simulink library "inp"  (R2021b)
settings: Solver=VariableStepAuto  StartTime=0.0  StopTime=10.0  RelTol=1e-3
undefined symbols (not defined in the file): C_TASK_5MS_S, FALSE, KINP_AcoreReadyToSlp_flg_ovrdflg, KINP_AcoreReadyToSlp_flg_ovrdval, KINP_AllowMovThd_OTA_enum_ovrdflg, KINP_AllowMovThd_OTA_enum_ovrdval, KINP_APSAngleTarget_Deg_ovrdflg, KINP_APSAngleTarget_Deg_ovrdval, KINP_APSDecReq_mps2_ovrdflg, KINP_APSDecReq_mps2_ovrdval, KINP_APSDecReqA_flg_ovrdflg, KINP_APSDecReqA_flg_ovrdval, KINP_APSDFLL_cm_ovrdflg, KINP_APSDFLL_cm_ovrdval, KINP_APSDFLR_cm_ovrdflg, KINP_APSDFLR_cm_ovrdval, KINP_APSDRLL_cm_ovrdflg, KINP_APSDRLL_cm_ovrdval, KINP_APSDRLR_cm_ovrdflg, KINP_APSDRLR_cm_ovrdval, KINP_APSExitCondition_enum_ovrdflg, KINP_APSExitCondition_enum_ovrdval, KINP_APSHWVer_enum_ovrdflg, KINP_APSHWVer_enum_ovrdval, KINP_APSProgressPCT_pct_ovrdflg, KINP_APSProgressPCT_pct_ovrdval, KINP_APSReq_enum_ovrdflg, KINP_APSReq_enum_ovrdval, KINP_APSRQDisplay_enum_ovrdflg, KINP_APSRQDisplay_enum_ovrdval, KINP_APSRqEPASCtrl_flg_ovrdflg, KINP_APSRqEPASCtrl_flg_ovrdval, KINP_APSShiftPosnReq_enum_ovrdval, KINP_APSShiftPosnReq_enum_ovrflg, KINP_APSSpeedCMD_kph_ovrdval, KINP_APSSpeedCMD_kph_ovrflg, KINP_APSStaSystem_enum_ovrdflg, KINP_APSStaSystem_enum_ovrdval, KINP_APSSWVer_enum_ovrdflg, KINP_APSSWVer_enum_ovrdval, KINP_APSVMCReqA_flg_ovrdval, KINP_APSVMCReqA_flg_ovrflg, KINP_APSVRqEPASCtrl_flg_ovrdflg, KINP_APSVRqEPASCtrl_flg_ovrdval, KINP_AuxBattVolmV_mV_ovrdflg, KINP_AuxBattVolmV_mV_ovrdval, KINP_CAASSta_enum_ovrdflg, KINP_CAASSta_enum_ovrdval, KINP_CAASVMCReqA_flg_ovrdval, KINP_CAASVMCReqA_flg_ovrflg, KINP_Chime_enum_ovrdflg, KINP_Chime_enum_ovrdval, KINP_ClearDTCcmd_flg_ovrdflg, KINP_ClearDTCcmd_flg_ovrdval, KINP_EvccAplusPwrUpReq_flg_ovrdflg, KINP_EvccAplusPwrUpReq_flg_ovrdval, KINP_LFID_raw_ovrdval, KINP_LFID_raw_ovrflg, KINP_LRID_raw_ovrdval, KINP_MemOffsetAccX_raw16_ovrdflg ... (+118)
libraries: FVT_lib x503, hcu_lib x1
(part 8 of 16)

== system inp/INP/CAN1/SignalCheck/EMC1_EM1 ==
  BHAL_outputs : Inport
  inp_CanValid_bus : Inport  Port=2
  EM1CS : FVT_lib/inp/can_signal_template  SystemSampleTime=-1  VariantActivationTime=update diagram  Latency=0  AutoFrameSizeCalculation=off
      link override defval: Value=KINP_EM1CS_enum_defval
      link override ovrdflg: Value=KINP_EM1CS_enum_ovrdflg
      link override ovrdval: Value=KINP_EM1CS_enum_ovrdval
  EM1Cnt : FVT_lib/inp/can_signal_template  SystemSampleTime=-1  VariantActivationTime=update diagram  Latency=0  AutoFrameSizeCalculation=off
      link override defval: Value=KINP_EM1Cnt_enum_defval
      link override ovrdflg: Value=KINP_EM1Cnt_enum_ovrdflg
      link override ovrdval: Value=KINP_EM1Cnt_enum_ovrdval
  EM1OvrCtrlMBrk : FVT_lib/inp/can_signal_template  SystemSampleTime=-1  VariantActivationTime=update diagram  Latency=0  AutoFrameSizeCalculation=off
      link override defval: Value=KINP_EM1OvrCtrlMBrk_enum_defval
      link override ovrdflg: Value=KINP_EM1OvrCtrlMBrk_enum_ovrdflg
      link override ovrdval: Value=KINP_EM1OvrCtrlMBrk_enum_ovrdval
  EM1OvrCtrlMDriv : FVT_lib/inp/can_signal_template  SystemSampleTime=-1  VariantActivationTime=update diagram  Latency=0  AutoFrameSizeCalculation=off
      link override defval: Value=KINP_EM1OvrCtrlMDriv_enum_defval
      link override ovrdflg: Value=KINP_EM1OvrCtrlMDriv_enum_ovrdflg
      link override ovrdval: Value=KINP_EM1OvrCtrlMDriv_enum_ovrdval
  EM1OvrCtrlMPriBrk : FVT_lib/inp/can_signal_template  SystemSampleTime=-1  VariantActivationTime=update diagram  Latency=0  AutoFrameSizeCalculation=off
      link override defval: Value=KINP_EM1OvrCtrlMPriBrk_enum_defval
      link override ovrdflg: Value=KINP_EM1OvrCtrlMPriBrk_enum_ovrdflg
      link override ovrdval: Value=KINP_EM1OvrCtrlMPriBrk_enum_ovrdval
  EM1OvrCtrlMPriDriv : FVT_lib/inp/can_signal_template  SystemSampleTime=-1  VariantActivationTime=update diagram  Latency=0  AutoFrameSizeCalculation=off
      link override defval: Value=KINP_EM1OvrCtrlMPriDriv_enum_defval
      link override ovrdflg: Value=KINP_EM1OvrCtrlMPriDriv_enum_ovrdflg
      link override ovrdval: Value=KINP_EM1OvrCtrlMPriDriv_enum_ovrdval
  EM1ReqTorqHRlsBrk : FVT_lib/inp/can_signal_template  SystemSampleTime=-1  VariantActivationTime=update diagram  Latency=0  AutoFrameSizeCalculation=off
      link override defval: Value=KINP_EM1ReqTorqHRlsBrk_pct_defval
      link override ovrdflg: Value=KINP_EM1ReqTorqHRlsBrk_pct_ovrdflg
      link override ovrdval: Value=KINP_EM1ReqTorqHRlsBrk_pct_ovrdval
  EM1ReqTorqHRlsDri : FVT_lib/inp/can_signal_template  SystemSampleTime=-1  VariantActivationTime=update diagram  Latency=0  AutoFrameSizeCalculation=off
      link override defval: Value=KINP_EM1ReqTorqHRlsDri_pct_defval
      link override ovrdflg: Value=KINP_EM1ReqTorqHRlsDri_pct_ovrdflg
      link override ovrdval: Value=KINP_EM1ReqTorqHRlsDri_pct_ovrdval
  EM1ReqTorqLimBrk : FVT_lib/inp/can_signal_template  SystemSampleTime=-1  VariantActivationTime=update diagram  Latency=0  AutoFrameSizeCalculation=off
      link override defval: Value=KINP_EM1ReqTorqLimBrk_pct_defval
      link override ovrdflg: Value=KINP_EM1ReqTorqLimBrk_pct_ovrdflg
      link override ovrdval: Value=KINP_EM1ReqTorqLimBrk_pct_ovrdval
  EM1ReqTorqLimDriv : FVT_lib/inp/can_signal_template  SystemSampleTime=-1  VariantActivationTime=update diagram  Latency=0  AutoFrameSizeCalculation=off
      link override defval: Value=KINP_EM1ReqTorqLimDriv_pct_defval
      link override ovrdflg: Value=KINP_EM1ReqTorqLimDriv_pct_ovrdflg
      link override ovrdval: Value=KINP_EM1ReqTorqLimDriv_pct_ovrdval
  Terminator_{1..10} (10 alike) : Terminator
  True_VHAL_EM1CS_enum : Constant  Value=TRUE  OutDataTypeStr=boolean
  True_VHAL_EM1Cnt_enum : Constant  Value=TRUE  OutDataTypeStr=boolean
  True_VHAL_EM1OvrCtrlMBrk_enum : Constant  Value=TRUE  OutDataTypeStr=boolean
  True_VHAL_EM1OvrCtrlMDriv_enum : Constant  Value=TRUE  OutDataTypeStr=boolean
  True_VHAL_EM1OvrCtrlMPriBrk_enum : Constant  Value=TRUE  OutDataTypeStr=boolean
  True_VHAL_EM1OvrCtrlMPriDriv_enum : Constant  Value=TRUE  OutDataTypeStr=boolean
  True_VHAL_EM1ReqTorqHRlsBrk_pct : Constant  Value=TRUE  OutDataTypeStr=boolean
  True_VHAL_EM1ReqTorqHRlsDri_pct : Constant  Value=TRUE  OutDataTypeStr=boolean
  True_VHAL_EM1ReqTorqLimBrk_pct : Constant  Value=TRUE  OutDataTypeStr=boolean
  True_VHAL_EM1ReqTorqLimDriv_pct : Constant  Value=TRUE  OutDataTypeStr=boolean
  slr1_{1..10} (10 alike) : BusSelector  OutputSignals=VINP_CANMsgValidEMC1EM1_flg
  slr_VHAL_EM1CS_enum : BusSelector  OutputSignals=VHAL_EM1CS_enum
  slr_VHAL_EM1Cnt_enum : BusSelector  OutputSignals=VHAL_EM1Cnt_enum
  slr_VHAL_EM1OvrCtrlMBrk_enum : BusSelector  OutputSignals=VHAL_EM1OvrCtrlMBrk_enum
  slr_VHAL_EM1OvrCtrlMDriv_enum : BusSelector  OutputSignals=VHAL_EM1OvrCtrlMDriv_enum
  slr_VHAL_EM1OvrCtrlMPriBrk_enum : BusSelector  OutputSignals=VHAL_EM1OvrCtrlMPriBrk_enum
  slr_VHAL_EM1OvrCtrlMPriDriv_enum : BusSelector  OutputSignals=VHAL_EM1OvrCtrlMPriDriv_enum
  slr_VHAL_EM1ReqTorqHRlsBrk_pct : BusSelector  OutputSignals=VHAL_EM1ReqTorqHRlsBrk_pct
  slr_VHAL_EM1ReqTorqHRlsDri_pct : BusSelector  OutputSignals=VHAL_EM1ReqTorqHRlsDri_pct
  slr_VHAL_EM1ReqTorqLimBrk_pct : BusSelector  OutputSignals=VHAL_EM1ReqTorqLimBrk_pct
  slr_VHAL_EM1ReqTorqLimDriv_pct : BusSelector  OutputSignals=VHAL_EM1ReqTorqLimDriv_pct
  VINP_EM1CS_enum : Outport
  VINP_EM1Cnt_enum : Outport  Port=2
  VINP_EM1OvrCtrlMBrk_enum : Outport  Port=3
  VINP_EM1OvrCtrlMDriv_enum : Outport  Port=4
  VINP_EM1OvrCtrlMPriBrk_enum : Outport  Port=5
  VINP_EM1OvrCtrlMPriDriv_enum : Outport  Port=6
  VINP_EM1ReqTorqHRlsBrk_pct : Outport  Port=7
  VINP_EM1ReqTorqHRlsDri_pct : Outport  Port=8
  VINP_EM1ReqTorqLimBrk_pct : Outport  Port=9
  VINP_EM1ReqTorqLimDriv_pct : Outport  Port=10
  wires:
  BHAL_outputs/1 -> [BHAL_outputs]
  inp_CanValid_bus/1 -> [inp_CanValid_bus]
  [BHAL_outputs] -> slr_VHAL_EM1CS_enum/1
  slr_VHAL_EM1CS_enum/1 -> EM1CS/1  "<VHAL_EM1CS_enum>"
  True_VHAL_EM1CS_enum/1 -> EM1CS/2
  [inp_CanValid_bus] -> slr1_1/1
  slr1_1/1 -> EM1CS/3  "<VINP_CANMsgValidEMC1EM1_flg>"
  EM1CS/1 -> VINP_EM1CS_enum/1  "VINP_EM1CS_enum"
  EM1CS/2 -> Terminator_1/1
  [BHAL_outputs] -> slr_VHAL_EM1Cnt_enum/1
  slr_VHAL_EM1Cnt_enum/1 -> EM1Cnt/1  "<VHAL_EM1Cnt_enum>"
  True_VHAL_EM1Cnt_enum/1 -> EM1Cnt/2
  [inp_CanValid_bus] -> slr1_2/1
  slr1_2/1 -> EM1Cnt/3  "<VINP_CANMsgValidEMC1EM1_flg>"
  EM1Cnt/1 -> VINP_EM1Cnt_enum/1  "VINP_EM1Cnt_enum"
  EM1Cnt/2 -> Terminator_2/1
  [BHAL_outputs] -> slr_VHAL_EM1OvrCtrlMBrk_enum/1
  slr_VHAL_EM1OvrCtrlMBrk_enum/1 -> EM1OvrCtrlMBrk/1  "<VHAL_EM1OvrCtrlMBrk_enum>"
  True_VHAL_EM1OvrCtrlMBrk_enum/1 -> EM1OvrCtrlMBrk/2
  [inp_CanValid_bus] -> slr1_3/1
  slr1_3/1 -> EM1OvrCtrlMBrk/3  "<VINP_CANMsgValidEMC1EM1_flg>"
  EM1OvrCtrlMBrk/1 -> VINP_EM1OvrCtrlMBrk_enum/1  "VINP_EM1OvrCtrlMBrk_enum"
  EM1OvrCtrlMBrk/2 -> Terminator_3/1
  [BHAL_outputs] -> slr_VHAL_EM1OvrCtrlMDriv_enum/1
  slr_VHAL_EM1OvrCtrlMDriv_enum/1 -> EM1OvrCtrlMDriv/1  "<VHAL_EM1OvrCtrlMDriv_enum>"
  True_VHAL_EM1OvrCtrlMDriv_enum/1 -> EM1OvrCtrlMDriv/2
  [inp_CanValid_bus] -> slr1_4/1
  slr1_4/1 -> EM1OvrCtrlMDriv/3  "<VINP_CANMsgValidEMC1EM1_flg>"
  EM1OvrCtrlMDriv/1 -> VINP_EM1OvrCtrlMDriv_enum/1  "VINP_EM1OvrCtrlMDriv_enum"
  EM1OvrCtrlMDriv/2 -> Terminator_4/1
  [BHAL_outputs] -> slr_VHAL_EM1OvrCtrlMPriBrk_enum/1
  slr_VHAL_EM1OvrCtrlMPriBrk_enum/1 -> EM1OvrCtrlMPriBrk/1  "<VHAL_EM1OvrCtrlMPriBrk_enum>"
  True_VHAL_EM1OvrCtrlMPriBrk_enum/1 -> EM1OvrCtrlMPriBrk/2
  [inp_CanValid_bus] -> slr1_5/1
  slr1_5/1 -> EM1OvrCtrlMPriBrk/3  "<VINP_CANMsgValidEMC1EM1_flg>"
  EM1OvrCtrlMPriBrk/1 -> VINP_EM1OvrCtrlMPriBrk_enum/1  "VINP_EM1OvrCtrlMPriBrk_enum"
  EM1OvrCtrlMPriBrk/2 -> Terminator_5/1
  [BHAL_outputs] -> slr_VHAL_EM1OvrCtrlMPriDriv_enum/1
  slr_VHAL_EM1OvrCtrlMPriDriv_enum/1 -> EM1OvrCtrlMPriDriv/1  "<VHAL_EM1OvrCtrlMPriDriv_enum>"
  True_VHAL_EM1OvrCtrlMPriDriv_enum/1 -> EM1OvrCtrlMPriDriv/2
  [inp_CanValid_bus] -> slr1_6/1
  slr1_6/1 -> EM1OvrCtrlMPriDriv/3  "<VINP_CANMsgValidEMC1EM1_flg>"
  EM1OvrCtrlMPriDriv/1 -> VINP_EM1OvrCtrlMPriDriv_enum/1  "VINP_EM1OvrCtrlMPriDriv_enum"
  EM1OvrCtrlMPriDriv/2 -> Terminator_6/1
  [BHAL_outputs] -> slr_VHAL_EM1ReqTorqHRlsBrk_pct/1
  slr_VHAL_EM1ReqTorqHRlsBrk_pct/1 -> EM1ReqTorqHRlsBrk/1  "<VHAL_EM1ReqTorqHRlsBrk_pct>"
  True_VHAL_EM1ReqTorqHRlsBrk_pct/1 -> EM1ReqTorqHRlsBrk/2
  [inp_CanValid_bus] -> slr1_7/1
  slr1_7/1 -> EM1ReqTorqHRlsBrk/3  "<VINP_CANMsgValidEMC1EM1_flg>"
  EM1ReqTorqHRlsBrk/1 -> VINP_EM1ReqTorqHRlsBrk_pct/1  "VINP_EM1ReqTorqHRlsBrk_pct"
  EM1ReqTorqHRlsBrk/2 -> Terminator_7/1
  [BHAL_outputs] -> slr_VHAL_EM1ReqTorqHRlsDri_pct/1
  slr_VHAL_EM1ReqTorqHRlsDri_pct/1 -> EM1ReqTorqHRlsDri/1  "<VHAL_EM1ReqTorqHRlsDri_pct>"
  True_VHAL_EM1ReqTorqHRlsDri_pct/1 -> EM1ReqTorqHRlsDri/2
  [inp_CanValid_bus] -> slr1_8/1
  slr1_8/1 -> EM1ReqTorqHRlsDri/3  "<VINP_CANMsgValidEMC1EM1_flg>"
  EM1ReqTorqHRlsDri/1 -> VINP_EM1ReqTorqHRlsDri_pct/1  "VINP_EM1ReqTorqHRlsDri_pct"
  EM1ReqTorqHRlsDri/2 -> Terminator_8/1
  [BHAL_outputs] -> slr_VHAL_EM1ReqTorqLimBrk_pct/1
  slr_VHAL_EM1ReqTorqLimBrk_pct/1 -> EM1ReqTorqLimBrk/1  "<VHAL_EM1ReqTorqLimBrk_pct>"
  True_VHAL_EM1ReqTorqLimBrk_pct/1 -> EM1ReqTorqLimBrk/2
  [inp_CanValid_bus] -> slr1_9/1
  slr1_9/1 -> EM1ReqTorqLimBrk/3  "<VINP_CANMsgValidEMC1EM1_flg>"
  EM1ReqTorqLimBrk/1 -> VINP_EM1ReqTorqLimBrk_pct/1  "VINP_EM1ReqTorqLimBrk_pct"
  EM1ReqTorqLimBrk/2 -> Terminator_9/1
  [BHAL_outputs] -> slr_VHAL_EM1ReqTorqLimDriv_pct/1
  slr_VHAL_EM1ReqTorqLimDriv_pct/1 -> EM1ReqTorqLimDriv/1  "<VHAL_EM1ReqTorqLimDriv_pct>"
  True_VHAL_EM1ReqTorqLimDriv_pct/1 -> EM1ReqTorqLimDriv/2
  [inp_CanValid_bus] -> slr1_10/1
  slr1_10/1 -> EM1ReqTorqLimDriv/3  "<VINP_CANMsgValidEMC1EM1_flg>"
  EM1ReqTorqLimDriv/1 -> VINP_EM1ReqTorqLimDriv_pct/1  "VINP_EM1ReqTorqLimDriv_pct"
  EM1ReqTorqLimDriv/2 -> Terminator_10/1

== system inp/INP/CAN1/SignalCheck/EPB1 ==
  BHAL_outputs : Inport
  inp_CanValid_bus : Inport  Port=2
  EPBParkingBrakeSta : FVT_lib/inp/can_signal_template  SystemSampleTime=-1  VariantActivationTime=update diagram  Latency=0  AutoFrameSizeCalculation=off
      link override defval: Value=KINP_EPBParkingBrakeSta_enum_defval
      link override ovrdflg: Value=KINP_EPBParkingBrakeSta_enum_ovrdflg
      link override ovrdval: Value=KINP_EPBParkingBrakeSta_enum_ovrdval
  Terminator_1 : Terminator
  True_VHAL_EPBParkingBrakeSta_enum : Constant  Value=TRUE  OutDataTypeStr=boolean
  slr1_1 : BusSelector  OutputSignals=VINP_CANMsgValidEPB1_flg
  slr_VHAL_EPBParkingBrakeSta_enum : BusSelector  OutputSignals=VHAL_EPBParkingBrakeSta_enum
  VINP_EPBParkingBrakeSta_enum : Outport
  wires:
  BHAL_outputs/1 -> [BHAL_outputs]
  inp_CanValid_bus/1 -> [inp_CanValid_bus]
  [BHAL_outputs] -> slr_VHAL_EPBParkingBrakeSta_enum/1
  slr_VHAL_EPBParkingBrakeSta_enum/1 -> EPBParkingBrakeSta/1  "<VHAL_EPBParkingBrakeSta_enum>"
  True_VHAL_EPBParkingBrakeSta_enum/1 -> EPBParkingBrakeSta/2
  [inp_CanValid_bus] -> slr1_1/1
  slr1_1/1 -> EPBParkingBrakeSta/3  "<VINP_CANMsgValidEPB1_flg>"
  EPBParkingBrakeSta/1 -> VINP_EPBParkingBrakeSta_enum/1  "VINP_EPBParkingBrakeSta_enum"
  EPBParkingBrakeSta/2 -> Terminator_1/1

== system inp/INP/CAN1/SignalCheck/PDU_Status_1 ==
  BHAL_outputs : Inport
  inp_CanValid_bus : Inport  Port=2
  PDUDCDCRlySta : FVT_lib/inp/can_signal_template  SystemSampleTime=-1  VariantActivationTime=update diagram  Latency=0  AutoFrameSizeCalculation=off
      link override defval: Value=KINP_PDUDCDCRlySta_enum_defval
      link override ovrdflg: Value=KINP_PDUDCDCRlySta_enum_ovrdflg
      link override ovrdval: Value=KINP_PDUDCDCRlySta_enum_ovrdval
  PDUEACRlySta : FVT_lib/inp/can_signal_template  SystemSampleTime=-1  VariantActivationTime=update diagram  Latency=0  AutoFrameSizeCalculation=off
      link override defval: Value=KINP_PDUEACRlySta_enum_defval
      link override ovrdflg: Value=KINP_PDUEACRlySta_enum_ovrdflg
      link override ovrdval: Value=KINP_PDUEACRlySta_enum_ovrdval
  PDUEHPSRlySta : FVT_lib/inp/can_signal_template  SystemSampleTime=-1  VariantActivationTime=update diagram  Latency=0  AutoFrameSizeCalculation=off
      link override defval: Value=KINP_PDUEHPSRlySta_enum_defval
      link override ovrdflg: Value=KINP_PDUEHPSRlySta_enum_ovrdflg
      link override ovrdval: Value=KINP_PDUEHPSRlySta_enum_ovrdval
  PDUSelfChkSta : FVT_lib/inp/can_signal_template  SystemSampleTime=-1  VariantActivationTime=update diagram  Latency=0  AutoFrameSizeCalculation=off
      link override defval: Value=KINP_PDUSelfChkSta_enum_defval
      link override ovrdflg: Value=KINP_PDUSelfChkSta_enum_ovrdflg
      link override ovrdval: Value=KINP_PDUSelfChkSta_enum_ovrdval
  Terminator_{1..4} (4 alike) : Terminator
  True_VHAL_PDUDCDCRlySta_enum : Constant  Value=TRUE  OutDataTypeStr=boolean
  True_VHAL_PDUEACRlySta_enum : Constant  Value=TRUE  OutDataTypeStr=boolean
  True_VHAL_PDUEHPSRlySta_enum : Constant  Value=TRUE  OutDataTypeStr=boolean
  True_VHAL_PDUSelfChkSta_enum : Constant  Value=TRUE  OutDataTypeStr=boolean
  slr1_{1..4} (4 alike) : BusSelector  OutputSignals=VINP_CANMsgValidPDUStatus1_flg
  slr_VHAL_PDUDCDCRlySta_enum : BusSelector  OutputSignals=VHAL_PDUDCDCRlySta_enum
  slr_VHAL_PDUEACRlySta_enum : BusSelector  OutputSignals=VHAL_PDUEACRlySta_enum
  slr_VHAL_PDUEHPSRlySta_enum : BusSelector  OutputSignals=VHAL_PDUEHPSRlySta_enum
  slr_VHAL_PDUSelfChkSta_enum : BusSelector  OutputSignals=VHAL_PDUSelfChkSta_enum
  VINP_PDUDCDCRlySta_enum : Outport
  VINP_PDUEACRlySta_enum : Outport  Port=2
  VINP_PDUEHPSRlySta_enum : Outport  Port=3
  VINP_PDUSelfChkSta_enum : Outport  Port=4
  wires:
  BHAL_outputs/1 -> [BHAL_outputs]
  inp_CanValid_bus/1 -> [inp_CanValid_bus]
  [BHAL_outputs] -> slr_VHAL_PDUDCDCRlySta_enum/1
  slr_VHAL_PDUDCDCRlySta_enum/1 -> PDUDCDCRlySta/1  "<VHAL_PDUDCDCRlySta_enum>"
  True_VHAL_PDUDCDCRlySta_enum/1 -> PDUDCDCRlySta/2
  [inp_CanValid_bus] -> slr1_1/1
  slr1_1/1 -> PDUDCDCRlySta/3  "<VINP_CANMsgValidPDUStatus1_flg>"
  PDUDCDCRlySta/1 -> VINP_PDUDCDCRlySta_enum/1  "VINP_PDUDCDCRlySta_enum"
  PDUDCDCRlySta/2 -> Terminator_1/1
  [BHAL_outputs] -> slr_VHAL_PDUEACRlySta_enum/1
  slr_VHAL_PDUEACRlySta_enum/1 -> PDUEACRlySta/1  "<VHAL_PDUEACRlySta_enum>"
  True_VHAL_PDUEACRlySta_enum/1 -> PDUEACRlySta/2
  [inp_CanValid_bus] -> slr1_2/1
  slr1_2/1 -> PDUEACRlySta/3  "<VINP_CANMsgValidPDUStatus1_flg>"
  PDUEACRlySta/1 -> VINP_PDUEACRlySta_enum/1  "VINP_PDUEACRlySta_enum"
  PDUEACRlySta/2 -> Terminator_2/1
  [BHAL_outputs] -> slr_VHAL_PDUEHPSRlySta_enum/1
  slr_VHAL_PDUEHPSRlySta_enum/1 -> PDUEHPSRlySta/1  "<VHAL_PDUEHPSRlySta_enum>"
  True_VHAL_PDUEHPSRlySta_enum/1 -> PDUEHPSRlySta/2
  [inp_CanValid_bus] -> slr1_3/1
  slr1_3/1 -> PDUEHPSRlySta/3  "<VINP_CANMsgValidPDUStatus1_flg>"
  PDUEHPSRlySta/1 -> VINP_PDUEHPSRlySta_enum/1  "VINP_PDUEHPSRlySta_enum"
  PDUEHPSRlySta/2 -> Terminator_3/1
  [BHAL_outputs] -> slr_VHAL_PDUSelfChkSta_enum/1
  slr_VHAL_PDUSelfChkSta_enum/1 -> PDUSelfChkSta/1  "<VHAL_PDUSelfChkSta_enum>"
  True_VHAL_PDUSelfChkSta_enum/1 -> PDUSelfChkSta/2
  [inp_CanValid_bus] -> slr1_4/1
  slr1_4/1 -> PDUSelfChkSta/3  "<VINP_CANMsgValidPDUStatus1_flg>"
  PDUSelfChkSta/1 -> VINP_PDUSelfChkSta_enum/1  "VINP_PDUSelfChkSta_enum"
  PDUSelfChkSta/2 -> Terminator_4/1

== system inp/INP/CAN2/SignalCheck/IVI1 ==
  BHAL_outputs : Inport
  inp_CanValid_bus : Inport  Port=2
  AmbLighLowBatAlertSW : FVT_lib/inp/can_signal_template  SystemSampleTime=-1  VariantActivationTime=update diagram  Latency=0  AutoFrameSizeCalculation=off
      link override defval: Value=KINP_AmbLighLowBatAlertSW_flg_defval
      link override ovrdflg: Value=KINP_AmbLighLowBatAlertSW_flg_ovrdflg
      link override ovrdval: Value=KINP_AmbLighLowBatAlertSW_flg_ovrdval
  AmbLighSafetyAlertSW : FVT_lib/inp/can_signal_template  SystemSampleTime=-1  VariantActivationTime=update diagram  Latency=0  AutoFrameSizeCalculation=off
      link override defval: Value=KINP_AmbLighSafetyAlertSW_flg_defval
      link override ovrdflg: Value=KINP_AmbLighSafetyAlertSW_flg_ovrdflg
      link override ovrdval: Value=KINP_AmbLighSafetyAlertSW_flg_ovrdval
  AmbLightColorSet : FVT_lib/inp/can_signal_template  SystemSampleTime=-1  VariantActivationTime=update diagram  Latency=0  AutoFrameSizeCalculation=off
      link override defval: Value=KINP_AmbLightColorSet_enum_defval
      link override ovrdflg: Value=KINP_AmbLightColorSet_enum_ovrdflg
      link override ovrdval: Value=KINP_AmbLightColorSet_enum_ovrdval
  AmbLightDimInDarkSW : FVT_lib/inp/can_signal_template  SystemSampleTime=-1  VariantActivationTime=update diagram  Latency=0  AutoFrameSizeCalculation=off
      link override defval: Value=KINP_AmbLightDimInDarkSW_flg_defval
      link override ovrdflg: Value=KINP_AmbLightDimInDarkSW_flg_ovrdflg
      link override ovrdval: Value=KINP_AmbLightDimInDarkSW_flg_ovrdval
  AmbLightSW : FVT_lib/inp/can_signal_template  SystemSampleTime=-1  VariantActivationTime=update diagram  Latency=0  AutoFrameSizeCalculation=off
      link override defval: Value=KINP_AmbLightSW_flg_defval
      link override ovrdflg: Value=KINP_AmbLightSW_flg_ovrdflg
      link override ovrdval: Value=KINP_AmbLightSW_flg_ovrdval
  AmbLightWlcmLightSW : FVT_lib/inp/can_signal_template  SystemSampleTime=-1  VariantActivationTime=update diagram  Latency=0  AutoFrameSizeCalculation=off
      link override defval: Value=KINP_AmbLightWlcmLightSW_flg_defval
      link override ovrdflg: Value=KINP_AmbLightWlcmLightSW_flg_ovrdflg
      link override ovrdval: Value=KINP_AmbLightWlcmLightSW_flg_ovrdval
  FCPFrEvtBtnACMaxReq : FVT_lib/inp/can_signal_template  SystemSampleTime=-1  VariantActivationTime=update diagram  Latency=0  AutoFrameSizeCalculation=off
      link override defval: Value=KINP_FCPFrEvtBtnACMaxReq_flg_defval
      link override ovrdflg: Value=KINP_FCPFrEvtBtnACMaxReq_flg_ovrdflg
      link override ovrdval: Value=KINP_FCPFrEvtBtnACMaxReq_flg_ovrdval
  FCPFrEvtBtnACReq : FVT_lib/inp/can_signal_template  SystemSampleTime=-1  VariantActivationTime=update diagram  Latency=0  AutoFrameSizeCalculation=off
      link override defval: Value=KINP_FCPFrEvtBtnACReq_flg_defval
      link override ovrdflg: Value=KINP_FCPFrEvtBtnACReq_flg_ovrdflg
      link override ovrdval: Value=KINP_FCPFrEvtBtnACReq_flg_ovrdval
  FCPFrEvtBtnAutoReq : FVT_lib/inp/can_signal_template  SystemSampleTime=-1  VariantActivationTime=update diagram  Latency=0  AutoFrameSizeCalculation=off
      link override defval: Value=KINP_FCPFrEvtBtnAutoReq_flg_defval
      link override ovrdflg: Value=KINP_FCPFrEvtBtnAutoReq_flg_ovrdflg
      link override ovrdval: Value=KINP_FCPFrEvtBtnAutoReq_flg_ovrdval
  FCPFrEvtBtnSyncReq : FVT_lib/inp/can_signal_template  SystemSampleTime=-1  VariantActivationTime=update diagram  Latency=0  AutoFrameSizeCalculation=off
      link override defval: Value=KINP_FCPFrEvtBtnSyncReq_flg_defval
      link override ovrdflg: Value=KINP_FCPFrEvtBtnSyncReq_flg_ovrdflg
      link override ovrdval: Value=KINP_FCPFrEvtBtnSyncReq_flg_ovrdval
  IVITimeCheck : FVT_lib/inp/can_signal_template  SystemSampleTime=-1  VariantActivationTime=update diagram  Latency=0  AutoFrameSizeCalculation=off
      link override defval: Value=KINP_IVITimeCheck_enum_defval
      link override ovrdflg: Value=KINP_IVITimeCheck_enum_ovrdflg
      link override ovrdval: Value=KINP_IVITimeCheck_enum_ovrdval
  IVITimeDay : FVT_lib/inp/can_signal_template  SystemSampleTime=-1  VariantActivationTime=update diagram  Latency=0  AutoFrameSizeCalculation=off
      link override defval: Value=KINP_IVITimeDay_DAY_defval
      link override ovrdflg: Value=KINP_IVITimeDay_DAY_ovrdflg
      link override ovrdval: Value=KINP_IVITimeDay_DAY_ovrdval
  IVITimeHour : FVT_lib/inp/can_signal_template  SystemSampleTime=-1  VariantActivationTime=update diagram  Latency=0  AutoFrameSizeCalculation=off
      link override defval: Value=KINP_IVITimeHour_hr_defval
      link override ovrdflg: Value=KINP_IVITimeHour_hr_ovrdflg
      link override ovrdval: Value=KINP_IVITimeHour_hr_ovrdval
  IVITimeMinute : FVT_lib/inp/can_signal_template  SystemSampleTime=-1  VariantActivationTime=update diagram  Latency=0  AutoFrameSizeCalculation=off
      link override defval: Value=KINP_IVITimeMinute_min_defval
      link override ovrdflg: Value=KINP_IVITimeMinute_min_ovrdflg
      link override ovrdval: Value=KINP_IVITimeMinute_min_ovrdval
  IVITimeMonth : FVT_lib/inp/can_signal_template  SystemSampleTime=-1  VariantActivationTime=update diagram  Latency=0  AutoFrameSizeCalculation=off
      link override defval: Value=KINP_IVITimeMonth_MONTH_defval
      link override ovrdflg: Value=KINP_IVITimeMonth_MONTH_ovrdflg
      link override ovrdval: Value=KINP_IVITimeMonth_MONTH_ovrdval
  IVITimeSecond : FVT_lib/inp/can_signal_template  SystemSampleTime=-1  VariantActivationTime=update diagram  Latency=0  AutoFrameSizeCalculation=off
      link override defval: Value=KINP_IVITimeSecond_s_defval
      link override ovrdflg: Value=KINP_IVITimeSecond_s_ovrdflg
      link override ovrdval: Value=KINP_IVITimeSecond_s_ovrdval
  IVITimeYear : FVT_lib/inp/can_signal_template  SystemSampleTime=-1  VariantActivationTime=update diagram  Latency=0  AutoFrameSizeCalculation=off
      link override defval: Value=KINP_IVITimeYear_YEAR_defval
      link override ovrdflg: Value=KINP_IVITimeYear_YEAR_ovrdflg
      link override ovrdval: Value=KINP_IVITimeYear_YEAR_ovrdval
  LINKtoDrive : FVT_lib/inp/can_signal_template  SystemSampleTime=-1  VariantActivationTime=update diagram  Latency=0  AutoFrameSizeCalculation=off
      link override defval: Value=KINP_LINKtoDrive_flg_defval
      link override ovrdflg: Value=KINP_LINKtoDrive_flg_ovrdflg
      link override ovrdval: Value=KINP_LINKtoDrive_flg_ovrdval
  OpenDrOpenWdoSW : FVT_lib/inp/can_signal_template  SystemSampleTime=-1  VariantActivationTime=update diagram  Latency=0  AutoFrameSizeCalculation=off
      link override defval: Value=KINP_OpenDrOpenWdoSW_flg_defval
      link override ovrdflg: Value=KINP_OpenDrOpenWdoSW_flg_ovrdflg
      link override ovrdval: Value=KINP_OpenDrOpenWdoSW_flg_ovrdval
  PWCONTINUEUSE : FVT_lib/inp/can_signal_template  SystemSampleTime=-1  VariantActivationTime=update diagram  Latency=0  AutoFrameSizeCalculation=off
      link override defval: Value=KINP_PWCONTINUEUSE_flg_defval
      link override ovrdflg: Value=KINP_PWCONTINUEUSE_flg_ovrdflg
      link override ovrdval: Value=KINP_PWCONTINUEUSE_flg_ovrdval
  SmartEcoModeSW : FVT_lib/inp/can_signal_template  SystemSampleTime=-1  VariantActivationTime=update diagram  Latency=0  AutoFrameSizeCalculation=off
      link override defval: Value=KINP_SmartEcoModeSW_flg_defval
      link override ovrdflg: Value=KINP_SmartEcoModeSW_flg_ovrdflg
      link override ovrdval: Value=KINP_SmartEcoModeSW_flg_ovrdval
  Terminator_{1..21} (21 alike) : Terminator
  True_VHAL_AmbLighLowBatAlertSW_flg : Constant  Value=TRUE  OutDataTypeStr=boolean
  True_VHAL_AmbLighSafetyAlertSW_flg : Constant  Value=TRUE  OutDataTypeStr=boolean
  True_VHAL_AmbLightColorSet_enum : Constant  Value=TRUE  OutDataTypeStr=boolean
  True_VHAL_AmbLightDimInDarkSW_flg : Constant  Value=TRUE  OutDataTypeStr=boolean
  True_VHAL_AmbLightSW_flg : Constant  Value=TRUE  OutDataTypeStr=boolean
  True_VHAL_AmbLightWlcmLightSW_flg : Constant  Value=TRUE  OutDataTypeStr=boolean
  True_VHAL_FCPFrEvtBtnACMaxReq_flg : Constant  Value=TRUE  OutDataTypeStr=boolean
  True_VHAL_FCPFrEvtBtnACReq_flg : Constant  Value=TRUE  OutDataTypeStr=boolean
  True_VHAL_FCPFrEvtBtnAutoReq_flg : Constant  Value=TRUE  OutDataTypeStr=boolean
  True_VHAL_FCPFrEvtBtnSyncReq_flg : Constant  Value=TRUE  OutDataTypeStr=boolean
  True_VHAL_IVITimeCheck_enum : Constant  Value=TRUE  OutDataTypeStr=boolean
  True_VHAL_IVITimeDay_DAY : Constant  Value=TRUE  OutDataTypeStr=boolean
  True_VHAL_IVITimeHour_hr : Constant  Value=TRUE  OutDataTypeStr=boolean
  True_VHAL_IVITimeMinute_min : Constant  Value=TRUE  OutDataTypeStr=boolean
  True_VHAL_IVITimeMonth_MONTH : Constant  Value=TRUE  OutDataTypeStr=boolean
  True_VHAL_IVITimeSecond_s : Constant  Value=TRUE  OutDataTypeStr=boolean
  True_VHAL_IVITimeYear_YEAR : Constant  Value=TRUE  OutDataTypeStr=boolean
  True_VHAL_LINKtoDrive_flg : Constant  Value=TRUE  OutDataTypeStr=boolean
  True_VHAL_OpenDrOpenWdoSW_flg : Constant  Value=TRUE  OutDataTypeStr=boolean
  True_VHAL_PWCONTINUEUSE_flg : Constant  Value=TRUE  OutDataTypeStr=boolean
  True_VHAL_SmartEcoModeSW_flg : Constant  Value=TRUE  OutDataTypeStr=boolean
  slr1_{1..21} (21 alike) : BusSelector  OutputSignals=VINP_CANMsgValidIVI1_flg
  slr_VHAL_AmbLighLowBatAlertSW_flg : BusSelector  OutputSignals=VHAL_AmbLighLowBatAlertSW_flg
  slr_VHAL_AmbLighSafetyAlertSW_flg : BusSelector  OutputSignals=VHAL_AmbLighSafetyAlertSW_flg
  slr_VHAL_AmbLightColorSet_enum : BusSelector  OutputSignals=VHAL_AmbLightColorSet_enum
  slr_VHAL_AmbLightDimInDarkSW_flg : BusSelector  OutputSignals=VHAL_AmbLightDimInDarkSW_flg
  slr_VHAL_AmbLightSW_flg : BusSelector  OutputSignals=VHAL_AmbLightSW_flg
  slr_VHAL_AmbLightWlcmLightSW_flg : BusSelector  OutputSignals=VHAL_AmbLightWlcmLightSW_flg
  slr_VHAL_FCPFrEvtBtnACMaxReq_flg : BusSelector  OutputSignals=VHAL_FCPFrEvtBtnACMaxReq_flg
  slr_VHAL_FCPFrEvtBtnACReq_flg : BusSelector  OutputSignals=VHAL_FCPFrEvtBtnACReq_flg
  slr_VHAL_FCPFrEvtBtnAutoReq_flg : BusSelector  OutputSignals=VHAL_FCPFrEvtBtnAutoReq_flg
  slr_VHAL_FCPFrEvtBtnSyncReq_flg : BusSelector  OutputSignals=VHAL_FCPFrEvtBtnSyncReq_flg
  slr_VHAL_IVITimeCheck_enum : BusSelector  OutputSignals=VHAL_IVITimeCheck_enum
  slr_VHAL_IVITimeDay_DAY : BusSelector  OutputSignals=VHAL_IVITimeDay_DAY
  slr_VHAL_IVITimeHour_hr : BusSelector  OutputSignals=VHAL_IVITimeHour_hr
  slr_VHAL_IVITimeMinute_min : BusSelector  OutputSignals=VHAL_IVITimeMinute_min
  slr_VHAL_IVITimeMonth_MONTH : BusSelector  OutputSignals=VHAL_IVITimeMonth_MONTH
  slr_VHAL_IVITimeSecond_s : BusSelector  OutputSignals=VHAL_IVITimeSecond_s
  slr_VHAL_IVITimeYear_YEAR : BusSelector  OutputSignals=VHAL_IVITimeYear_YEAR
  slr_VHAL_LINKtoDrive_flg : BusSelector  OutputSignals=VHAL_LINKtoDrive_flg
  slr_VHAL_OpenDrOpenWdoSW_flg : BusSelector  OutputSignals=VHAL_OpenDrOpenWdoSW_flg
  slr_VHAL_PWCONTINUEUSE_flg : BusSelector  OutputSignals=VHAL_PWCONTINUEUSE_flg
  slr_VHAL_SmartEcoModeSW_flg : BusSelector  OutputSignals=VHAL_SmartEcoModeSW_flg
  VINP_AmbLighLowBatAlertSW_flg : Outport
  VINP_AmbLighSafetyAlertSW_flg : Outport  Port=2
  VINP_AmbLightColorSet_enum : Outport  Port=3
  VINP_AmbLightDimInDarkSW_flg : Outport  Port=4
  VINP_AmbLightSW_flg : Outport  Port=5
  VINP_AmbLightWlcmLightSW_flg : Outport  Port=6
  VINP_FCPFrEvtBtnACMaxReq_flg : Outport  Port=7
  VINP_FCPFrEvtBtnACReq_flg : Outport  Port=8
  VINP_FCPFrEvtBtnAutoReq_flg : Outport  Port=9
  VINP_FCPFrEvtBtnSyncReq_flg : Outport  Port=10
  VINP_IVITimeCheck_enum : Outport  Port=11
  VINP_IVITimeDay_DAY : Outport  Port=12
  VINP_IVITimeHour_hr : Outport  Port=13
  VINP_IVITimeMinute_min : Outport  Port=14
  VINP_IVITimeMonth_MONTH : Outport  Port=15
  VINP_IVITimeSecond_s : Outport  Port=16
  VINP_IVITimeYear_YEAR : Outport  Port=17
  VINP_LINKtoDrive_flg : Outport  Port=18
  VINP_OpenDrOpenWdoSW_flg : Outport  Port=19
  VINP_PWCONTINUEUSE_flg : Outport  Port=20
  VINP_SmartEcoModeSW_flg : Outport  Port=21
  wires:
  BHAL_outputs/1 -> [BHAL_outputs]
  inp_CanValid_bus/1 -> [inp_CanValid_bus]
  [BHAL_outputs] -> slr_VHAL_AmbLighLowBatAlertSW_flg/1
  slr_VHAL_AmbLighLowBatAlertSW_flg/1 -> AmbLighLowBatAlertSW/1  "<VHAL_AmbLighLowBatAlertSW_flg>"
  True_VHAL_AmbLighLowBatAlertSW_flg/1 -> AmbLighLowBatAlertSW/2
  [inp_CanValid_bus] -> slr1_1/1
  slr1_1/1 -> AmbLighLowBatAlertSW/3  "<VINP_CANMsgValidIVI1_flg>"
  AmbLighLowBatAlertSW/1 -> VINP_AmbLighLowBatAlertSW_flg/1  "VINP_AmbLighLowBatAlertSW_flg"
  AmbLighLowBatAlertSW/2 -> Terminator_1/1
  [BHAL_outputs] -> slr_VHAL_AmbLighSafetyAlertSW_flg/1
  slr_VHAL_AmbLighSafetyAlertSW_flg/1 -> AmbLighSafetyAlertSW/1  "<VHAL_AmbLighSafetyAlertSW_flg>"
  True_VHAL_AmbLighSafetyAlertSW_flg/1 -> AmbLighSafetyAlertSW/2
  [inp_CanValid_bus] -> slr1_2/1
  slr1_2/1 -> AmbLighSafetyAlertSW/3  "<VINP_CANMsgValidIVI1_flg>"
  AmbLighSafetyAlertSW/1 -> VINP_AmbLighSafetyAlertSW_flg/1  "VINP_AmbLighSafetyAlertSW_flg"
  AmbLighSafetyAlertSW/2 -> Terminator_2/1
  [BHAL_outputs] -> slr_VHAL_AmbLightColorSet_enum/1
  slr_VHAL_AmbLightColorSet_enum/1 -> AmbLightColorSet/1  "<VHAL_AmbLightColorSet_enum>"
  True_VHAL_AmbLightColorSet_enum/1 -> AmbLightColorSet/2
  [inp_CanValid_bus] -> slr1_3/1
  slr1_3/1 -> AmbLightColorSet/3  "<VINP_CANMsgValidIVI1_flg>"
  AmbLightColorSet/1 -> VINP_AmbLightColorSet_enum/1  "VINP_AmbLightColorSet_enum"
  AmbLightColorSet/2 -> Terminator_3/1
  [BHAL_outputs] -> slr_VHAL_AmbLightDimInDarkSW_flg/1
  slr_VHAL_AmbLightDimInDarkSW_flg/1 -> AmbLightDimInDarkSW/1  "<VHAL_AmbLightDimInDarkSW_flg>"
  True_VHAL_AmbLightDimInDarkSW_flg/1 -> AmbLightDimInDarkSW/2
  [inp_CanValid_bus] -> slr1_4/1
  slr1_4/1 -> AmbLightDimInDarkSW/3  "<VINP_CANMsgValidIVI1_flg>"
  AmbLightDimInDarkSW/1 -> VINP_AmbLightDimInDarkSW_flg/1  "VINP_AmbLightDimInDarkSW_flg"
  AmbLightDimInDarkSW/2 -> Terminator_4/1
  [BHAL_outputs] -> slr_VHAL_AmbLightSW_flg/1
  slr_VHAL_AmbLightSW_flg/1 -> AmbLightSW/1  "<VHAL_AmbLightSW_flg>"
  True_VHAL_AmbLightSW_flg/1 -> AmbLightSW/2
  [inp_CanValid_bus] -> slr1_5/1
  slr1_5/1 -> AmbLightSW/3  "<VINP_CANMsgValidIVI1_flg>"
  AmbLightSW/1 -> VINP_AmbLightSW_flg/1  "VINP_AmbLightSW_flg"
  AmbLightSW/2 -> Terminator_5/1
  [BHAL_outputs] -> slr_VHAL_AmbLightWlcmLightSW_flg/1
  slr_VHAL_AmbLightWlcmLightSW_flg/1 -> AmbLightWlcmLightSW/1  "<VHAL_AmbLightWlcmLightSW_flg>"
  True_VHAL_AmbLightWlcmLightSW_flg/1 -> AmbLightWlcmLightSW/2
  [inp_CanValid_bus] -> slr1_6/1
  slr1_6/1 -> AmbLightWlcmLightSW/3  "<VINP_CANMsgValidIVI1_flg>"
  AmbLightWlcmLightSW/1 -> VINP_AmbLightWlcmLightSW_flg/1  "VINP_AmbLightWlcmLightSW_flg"
  AmbLightWlcmLightSW/2 -> Terminator_6/1
  [BHAL_outputs] -> slr_VHAL_FCPFrEvtBtnACMaxReq_flg/1
  slr_VHAL_FCPFrEvtBtnACMaxReq_flg/1 -> FCPFrEvtBtnACMaxReq/1  "<VHAL_FCPFrEvtBtnACMaxReq_flg>"
  True_VHAL_FCPFrEvtBtnACMaxReq_flg/1 -> FCPFrEvtBtnACMaxReq/2
  [inp_CanValid_bus] -> slr1_7/1
  slr1_7/1 -> FCPFrEvtBtnACMaxReq/3  "<VINP_CANMsgValidIVI1_flg>"
  FCPFrEvtBtnACMaxReq/1 -> VINP_FCPFrEvtBtnACMaxReq_flg/1  "VINP_FCPFrEvtBtnACMaxReq_flg"
  FCPFrEvtBtnACMaxReq/2 -> Terminator_7/1
  [BHAL_outputs] -> slr_VHAL_FCPFrEvtBtnACReq_flg/1
  slr_VHAL_FCPFrEvtBtnACReq_flg/1 -> FCPFrEvtBtnACReq/1  "<VHAL_FCPFrEvtBtnACReq_flg>"
  True_VHAL_FCPFrEvtBtnACReq_flg/1 -> FCPFrEvtBtnACReq/2
  [inp_CanValid_bus] -> slr1_8/1
  slr1_8/1 -> FCPFrEvtBtnACReq/3  "<VINP_CANMsgValidIVI1_flg>"
  FCPFrEvtBtnACReq/1 -> VINP_FCPFrEvtBtnACReq_flg/1  "VINP_FCPFrEvtBtnACReq_flg"
  FCPFrEvtBtnACReq/2 -> Terminator_8/1
  [BHAL_outputs] -> slr_VHAL_FCPFrEvtBtnAutoReq_flg/1
  slr_VHAL_FCPFrEvtBtnAutoReq_flg/1 -> FCPFrEvtBtnAutoReq/1  "<VHAL_FCPFrEvtBtnAutoReq_flg>"
  True_VHAL_FCPFrEvtBtnAutoReq_flg/1 -> FCPFrEvtBtnAutoReq/2
  [inp_CanValid_bus] -> slr1_9/1
  slr1_9/1 -> FCPFrEvtBtnAutoReq/3  "<VINP_CANMsgValidIVI1_flg>"
  FCPFrEvtBtnAutoReq/1 -> VINP_FCPFrEvtBtnAutoReq_flg/1  "VINP_FCPFrEvtBtnAutoReq_flg"
  FCPFrEvtBtnAutoReq/2 -> Terminator_9/1
  [BHAL_outputs] -> slr_VHAL_FCPFrEvtBtnSyncReq_flg/1
  slr_VHAL_FCPFrEvtBtnSyncReq_flg/1 -> FCPFrEvtBtnSyncReq/1  "<VHAL_FCPFrEvtBtnSyncReq_flg>"
  True_VHAL_FCPFrEvtBtnSyncReq_flg/1 -> FCPFrEvtBtnSyncReq/2
  [inp_CanValid_bus] -> slr1_10/1
  slr1_10/1 -> FCPFrEvtBtnSyncReq/3  "<VINP_CANMsgValidIVI1_flg>"
  FCPFrEvtBtnSyncReq/1 -> VINP_FCPFrEvtBtnSyncReq_flg/1  "VINP_FCPFrEvtBtnSyncReq_flg"
  FCPFrEvtBtnSyncReq/2 -> Terminator_10/1
  [BHAL_outputs] -> slr_VHAL_IVITimeCheck_enum/1
  slr_VHAL_IVITimeCheck_enum/1 -> IVITimeCheck/1  "<VHAL_IVITimeCheck_enum>"
  True_VHAL_IVITimeCheck_enum/1 -> IVITimeCheck/2
  [inp_CanValid_bus] -> slr1_11/1
  slr1_11/1 -> IVITimeCheck/3  "<VINP_CANMsgValidIVI1_flg>"
  IVITimeCheck/1 -> VINP_IVITimeCheck_enum/1  "VINP_IVITimeCheck_enum"
  IVITimeCheck/2 -> Terminator_11/1
  [BHAL_outputs] -> slr_VHAL_IVITimeDay_DAY/1
  slr_VHAL_IVITimeDay_DAY/1 -> IVITimeDay/1  "<VHAL_IVITimeDay_DAY>"
  True_VHAL_IVITimeDay_DAY/1 -> IVITimeDay/2
  [inp_CanValid_bus] -> slr1_12/1
  slr1_12/1 -> IVITimeDay/3  "<VINP_CANMsgValidIVI1_flg>"
  IVITimeDay/1 -> VINP_IVITimeDay_DAY/1  "VINP_IVITimeDay_DAY"
  IVITimeDay/2 -> Terminator_12/1
  [BHAL_outputs] -> slr_VHAL_IVITimeHour_hr/1
  slr_VHAL_IVITimeHour_hr/1 -> IVITimeHour/1  "<VHAL_IVITimeHour_hr>"
  True_VHAL_IVITimeHour_hr/1 -> IVITimeHour/2
  [inp_CanValid_bus] -> slr1_13/1
  slr1_13/1 -> IVITimeHour/3  "<VINP_CANMsgValidIVI1_flg>"
  IVITimeHour/1 -> VINP_IVITimeHour_hr/1  "VINP_IVITimeHour_hr"
  IVITimeHour/2 -> Terminator_13/1
  [BHAL_outputs] -> slr_VHAL_IVITimeMinute_min/1
  slr_VHAL_IVITimeMinute_min/1 -> IVITimeMinute/1  "<VHAL_IVITimeMinute_min>"
  True_VHAL_IVITimeMinute_min/1 -> IVITimeMinute/2
  [inp_CanValid_bus] -> slr1_14/1
  slr1_14/1 -> IVITimeMinute/3  "<VINP_CANMsgValidIVI1_flg>"
  IVITimeMinute/1 -> VINP_IVITimeMinute_min/1  "VINP_IVITimeMinute_min"
  IVITimeMinute/2 -> Terminator_14/1
  [BHAL_outputs] -> slr_VHAL_IVITimeMonth_MONTH/1
  slr_VHAL_IVITimeMonth_MONTH/1 -> IVITimeMonth/1  "<VHAL_IVITimeMonth_MONTH>"
  True_VHAL_IVITimeMonth_MONTH/1 -> IVITimeMonth/2
  [inp_CanValid_bus] -> slr1_15/1
  slr1_15/1 -> IVITimeMonth/3  "<VINP_CANMsgValidIVI1_flg>"
  IVITimeMonth/1 -> VINP_IVITimeMonth_MONTH/1  "VINP_IVITimeMonth_MONTH"
  IVITimeMonth/2 -> Terminator_15/1
  [BHAL_outputs] -> slr_VHAL_IVITimeSecond_s/1
  slr_VHAL_IVITimeSecond_s/1 -> IVITimeSecond/1  "<VHAL_IVITimeSecond_s>"
  True_VHAL_IVITimeSecond_s/1 -> IVITimeSecond/2
  [inp_CanValid_bus] -> slr1_16/1
  slr1_16/1 -> IVITimeSecond/3  "<VINP_CANMsgValidIVI1_flg>"
  IVITimeSecond/1 -> VINP_IVITimeSecond_s/1  "VINP_IVITimeSecond_s"
  IVITimeSecond/2 -> Terminator_16/1
  [BHAL_outputs] -> slr_VHAL_IVITimeYear_YEAR/1
  slr_VHAL_IVITimeYear_YEAR/1 -> IVITimeYear/1  "<VHAL_IVITimeYear_YEAR>"
  True_VHAL_IVITimeYear_YEAR/1 -> IVITimeYear/2
  [inp_CanValid_bus] -> slr1_17/1
  slr1_17/1 -> IVITimeYear/3  "<VINP_CANMsgValidIVI1_flg>"
  IVITimeYear/1 -> VINP_IVITimeYear_YEAR/1  "VINP_IVITimeYear_YEAR"
  IVITimeYear/2 -> Terminator_17/1
  [BHAL_outputs] -> slr_VHAL_LINKtoDrive_flg/1
  slr_VHAL_LINKtoDrive_flg/1 -> LINKtoDrive/1  "<VHAL_LINKtoDrive_flg>"
  True_VHAL_LINKtoDrive_flg/1 -> LINKtoDrive/2
  [inp_CanValid_bus] -> slr1_18/1
  slr1_18/1 -> LINKtoDrive/3  "<VINP_CANMsgValidIVI1_flg>"
  LINKtoDrive/1 -> VINP_LINKtoDrive_flg/1  "VINP_LINKtoDrive_flg"
  LINKtoDrive/2 -> Terminator_18/1
  [BHAL_outputs] -> slr_VHAL_OpenDrOpenWdoSW_flg/1
  slr_VHAL_OpenDrOpenWdoSW_flg/1 -> OpenDrOpenWdoSW/1  "<VHAL_OpenDrOpenWdoSW_flg>"
  True_VHAL_OpenDrOpenWdoSW_flg/1 -> OpenDrOpenWdoSW/2
  [inp_CanValid_bus] -> slr1_19/1
  slr1_19/1 -> OpenDrOpenWdoSW/3  "<VINP_CANMsgValidIVI1_flg>"
  OpenDrOpenWdoSW/1 -> VINP_OpenDrOpenWdoSW_flg/1  "VINP_OpenDrOpenWdoSW_flg"
  OpenDrOpenWdoSW/2 -> Terminator_19/1
  [BHAL_outputs] -> slr_VHAL_PWCONTINUEUSE_flg/1
  slr_VHAL_PWCONTINUEUSE_flg/1 -> PWCONTINUEUSE/1  "<VHAL_PWCONTINUEUSE_flg>"
  True_VHAL_PWCONTINUEUSE_flg/1 -> PWCONTINUEUSE/2
  [inp_CanValid_bus] -> slr1_20/1
  slr1_20/1 -> PWCONTINUEUSE/3  "<VINP_CANMsgValidIVI1_flg>"
  PWCONTINUEUSE/1 -> VINP_PWCONTINUEUSE_flg/1  "VINP_PWCONTINUEUSE_flg"
  PWCONTINUEUSE/2 -> Terminator_20/1
  [BHAL_outputs] -> slr_VHAL_SmartEcoModeSW_flg/1
  slr_VHAL_SmartEcoModeSW_flg/1 -> SmartEcoModeSW/1  "<VHAL_SmartEcoModeSW_flg>"
  True_VHAL_SmartEcoModeSW_flg/1 -> SmartEcoModeSW/2
  [inp_CanValid_bus] -> slr1_21/1
  slr1_21/1 -> SmartEcoModeSW/3  "<VINP_CANMsgValidIVI1_flg>"
  SmartEcoModeSW/1 -> VINP_SmartEcoModeSW_flg/1  "VINP_SmartEcoModeSW_flg"
  SmartEcoModeSW/2 -> Terminator_21/1
